simulink model "Longitudinal_old"  (R2025b)
settings: Solver=VariableStepAuto  StartTime=0.0  StopTime=100  RelTol=1e-3
undefined symbols (not defined in the file): car, m, R, Tau_1, Tau_2, Tau_3, Tau_4, Tau_EM, tyre
libraries: simulink x4
(part 1 of 2)
settings Model: Creator=mzacc  LastModifiedBy=giust

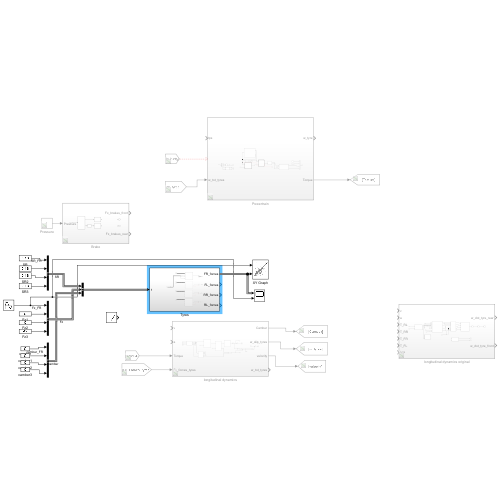
[thumbnail: Simulink's stored preview of the top-level diagram]
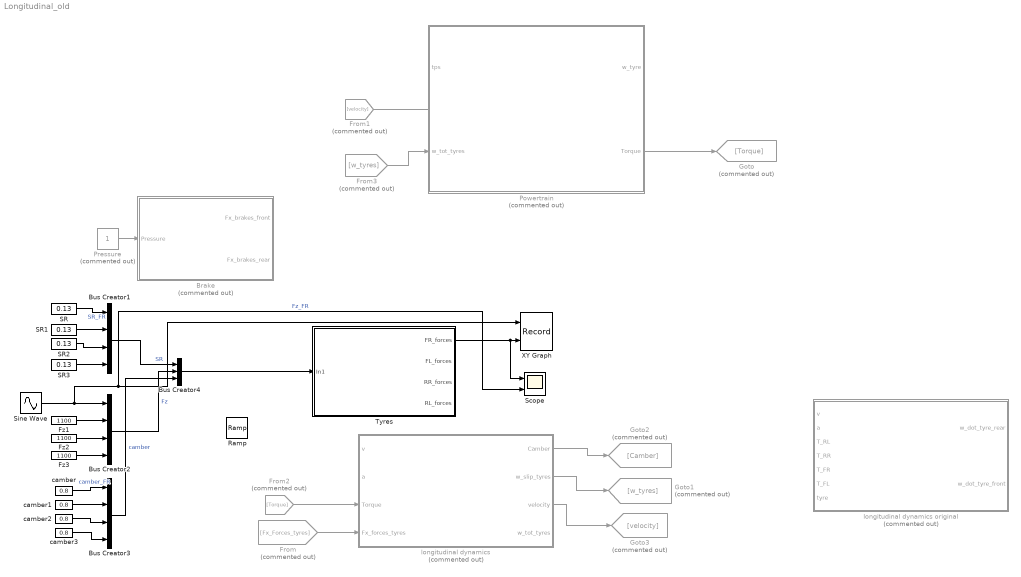
== system Longitudinal_old ==
  Brake : Subsystem  Commented=on
  Bus Creator1 : BusCreator  Inputs=4
  Bus Creator2 : BusCreator  Inputs=4
  Bus Creator3 : BusCreator  Inputs=4
  Bus Creator4 : BusCreator  Inputs=3
  From : From  Commented=on  GotoTag=Fx_Forces_tyres
  From1 : From  Commented=on  GotoTag=velocity
  From2 : From  Commented=on  GotoTag=Torque
  From3 : From  Commented=on  GotoTag=w_tyres
  Fz1 : Constant  Value=1100
  Fz2 : Constant  Value=1100
  Fz3 : Constant  Value=1100
  Goto : Goto  Commented=on  GotoTag=Torque
  Goto1 : Goto  Commented=on  GotoTag=w_tyres
  Goto2 : Goto  Commented=on  GotoTag=Camber
  Goto3 : Goto  Commented=on  GotoTag=velocity
  Powertrain : Subsystem  Commented=on
  Pressure : Constant  Commented=on
  Ramp : simulink/Sources/Ramp  slope=0.05  start=0  InitialOutput=-3
  SR{,1..3} (4 alike) : Constant  Value=0.13
  Scope : Scope  NumInputPorts=2
      settings: ActiveDisplayYMinimum=-298.14658012826334  ActiveDisplayYMaximum=2683.3192211543706
  Sine Wave : Sin  Amplitude=550  Bias=550  SampleTime=0
  Tyres : Subsystem
  XY Graph : Record  NumPorts=2.0  FileSettingsInternal="{\"entries\":[{\"content\":{\"excelSettings\":{\"content\":{},\"type\":\"Streamout.ExcelSettings\"},\"parquetSettings\":{\"content\":{},\"type\":\"Streamout.ParquetSettings\"}},\"type\":\"Streamout.FileSettingStorage\",\"uuid\":\"\"}],\"packageUris\":[\"http:\\/\\/schema.mathworks.com\\/mf0\\/streamout_blocks\\/R2020a\"],\"version\":\"1.0\"}"  FrameSettings=[0, 0]  Layout=[1 1]  SignalsInternal="{\"entries\":[{\"content\":{\"signals\":[{\"content\":{\"blockPath\":[],\"dimensions\":[1],\"domain\":\"\",\"lineColor\":\"#a2142f\",\"plots\":[ 1 ],\"port\":1,\"sid\":[\"\"],\"signalID\":1,\"signalName\":\"Fz_FR\"},\"type\":\"RecordBlkView.Signal\",\"uuid\":\"\"},{\"content\":{\"blockPath\":[],\"dimensions\":[1],\"domain\":\"\",\"hasChildren\":true,\"lineColor\":\"#4dbeee\",\"lineWidth\":2,\"port\":2,\"sid\":[\"\"],\"signalID\":2,\"signalName\":\"Tyres:1\"},\"type\":\"RecordBlkView.Signal\",\"uuid\":\"\"},{\"content\":{\"blockPath\":[],\"dimensions\":[1],\"domain\":\"\",\"leafPath\":\"Tyres:1.Fx_FR\",\"lineColor\":\"#7e2f8e\",\"lineWidth\":2,\"parentID\":2,\"plots\":[ 1 ],\"port\":2,\"sid\":[\"\"],\"signalID\":3,\"signalName\":\"Tyres:1.Fx_FR\"},\"type\":\"RecordBlkView.Signal\",\"uuid\":\"\"},{\"content\":{\"blockPath\":[],\"dimensions\":[1],\"domain\":\"\",\"leafPath\":\"Tyres:1.signal2\",\"lineColor\":\"#b746ff\",\"lineWidth\":2,\"parentID\":2,\"port\":2,\"sid\":[\"\"],\"signalID\":4,\"signalName\":\"Tyres:1.signal2\"},\"type\":\"RecordBlkView.Signal\",\"uuid\":\"\"}]},\"type\":\"RecordBlkView.InputSignals\",\"uuid\":\"\"}],\"packageUris\":[\"http:\\/\\/schema.mathworks.com\\/mf0\\/streamout_blocks\\/R2020a\"],\"version\":\"1.0\"}"  VisualizationBindings="{\"xyplotplugin\":{\"info\":[{\"series\":[{\"bindingParametersList\":[{\"parameter\":\"X-Axis\",\"signalID\":1,\"signalName\":\"Fz_FR\"},{\"parameter\":\"Y-Axis\",\"signalID\":3,\"signalName\":\"Tyres:1.Fx_FR\"},{\"parameter\":\"X-Axis\",\"signalID\":1,\"signalName\":\"Fz_FR\"},{\"parameter\":\"Y-Axis\",\"signalID\":3,\"signalName\":\"Tyres:1.Fx_FR\"}],\"seriesID\":0}],\"subplotID\":1}]}}"  CompatibilityTag=XY
  camber{,1..3} (4 alike) : Constant  Value=0.8
  longitudinal dynamics : Subsystem  Commented=on
  longitudinal dynamics original : Subsystem  Commented=on
  wires:
  Pressure/1 -> Brake/1(Pressure)
  From/1 -> longitudinal dynamics/4(Fx_forces_tyres)
  From2/1 -> longitudinal dynamics/3(Torque)
  Powertrain/2(Torque) -> Goto/1
  longitudinal dynamics/2(w_slip_tyres) -> Goto1/1
  longitudinal dynamics/1(Camber) -> Goto2/1
  longitudinal dynamics/3(velocity) -> Goto3/1
  From1/1 -> ?
  From3/1 -> Powertrain/2(w_tot_tyres)
  SR/1 -> Bus Creator1/1  "SR_FR"
  SR1/1 -> Bus Creator1/2
  SR2/1 -> Bus Creator1/3
  SR3/1 -> Bus Creator1/4
  Sine Wave/1 -> Scope/2, XY Graph/1, Bus Creator2/1  "Fz_FR"
  Fz1/1 -> Bus Creator2/2
  Fz2/1 -> Bus Creator2/3
  Fz3/1 -> Bus Creator2/4
  camber/1 -> Bus Creator3/1  "camber_FR"
  camber1/1 -> Bus Creator3/2
  camber2/1 -> Bus Creator3/3
  camber3/1 -> Bus Creator3/4
  Bus Creator1/1 -> Bus Creator4/1  "SR"
  Bus Creator2/1 -> Bus Creator4/2  "Fz"
  Bus Creator3/1 -> Bus Creator4/3  "camber"
  Bus Creator4/1 -> Tyres/1(In1)
  Tyres/1(FR_forces) -> Scope/1, XY Graph/2

== system Longitudinal_old/Brake ==
  Pressure : Inport
  Brake Balance : Subsystem
  Front Caliper : Subsystem
  Proportioning Valve : Subsystem
  Rear Caliper : Subsystem
  Fx_brakes_front : Outport
  Fx_brakes_rear : Outport  Port=2
  wires:
  Pressure/1 -> Brake Balance/1(In1)
  Brake Balance/1(P_Front) -> Front Caliper/1(P_Front)
  Proportioning Valve/1(p_rear_mod) -> Rear Caliper/1(P_rear)
  Brake Balance/2(P_rear) -> Proportioning Valve/1(P_rear)

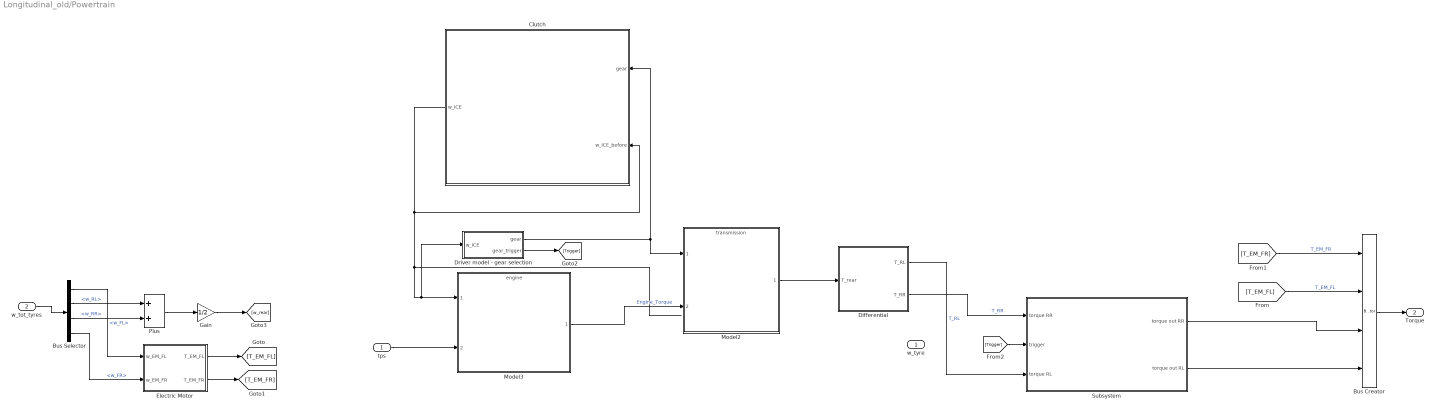
== system Longitudinal_old/Powertrain ==
  tps : Inport
  w_tot_tyres : Inport  Port=2
  Bus Creator : BusCreator  Inputs=4
  Bus Selector : BusSelector  OutputSignals=w_FL,w_RL,w_RR,w_FR
  Clutch : Subsystem
  Differential : Subsystem
  Driver model - gear selection : Subsystem
  Electric Motor : Subsystem
  Gain : Gain  Gain=1/2
  Model2 : ModelReference  ModelNameDialog=transmission.slx  SimulationMode=Normal  ModelReferenceVersion=3.9
  Model3 : ModelReference  ModelNameDialog=engine.slx  SimulationMode=Normal  ModelReferenceVersion=3.1
  Plus : Sum
  Subsystem : Subsystem
  w_tyre : Outport
  Torque : Outport  Port=2
  wires:
  Model3/1 -> Model2/2  "Engine_Torque"
  tps/1 -> Model3/2
  Model2/1 -> Differential/1(T_rear)
  ? -> w_tyre/1
  Bus Creator/1 -> Torque/1
  Electric Motor/1(T_EM_FL) -> [T_EM_FL]
  Electric Motor/2(T_EM_FR) -> [T_EM_FR]
  [T_EM_FL] -> Bus Creator/2  "T_EM_FL"
  [T_EM_FR] -> Bus Creator/1  "T_EM_FR"
  Differential/2(T_RR) -> Subsystem/1(torque RR)  "T_RR"
  Differential/1(T_RL) -> Subsystem/3(torque RL)  "T_RL"
  Subsystem/1(torque out RR) -> Bus Creator/3
  Subsystem/2(torque out RL) -> Bus Creator/4
  Driver model - gear selection/2(gear_trigger) -> [Trigger]
  [Trigger] -> Subsystem/2(trigger)
  w_tot_tyres/1 -> Bus Selector/1
  Bus Selector/1 -> Electric Motor/1(w_EM_FL)  "<w_FL>"
  Bus Selector/2 -> Plus/1  "<w_RL>"
  Bus Selector/4 -> Electric Motor/2(w_EM_FR)  "<w_FR>"
  Gain/1 -> [w_rear]
  Bus Selector/3 -> Plus/2  "<w_RR>"
  Plus/1 -> Gain/1
  Driver model - gear selection/1(gear) -> Clutch/1(gear), Model2/1
  Clutch/1(w_ICE) -> Clutch/2(w_ICE_before), Model3/1, Driver model - gear selection/1(w_ICE)

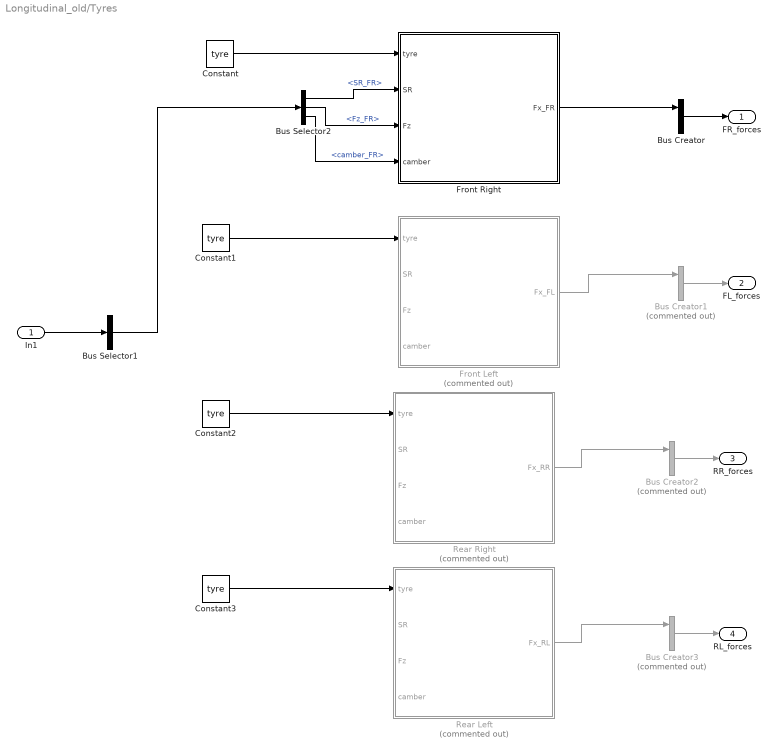
== system Longitudinal_old/Tyres ==
  In1 : Inport
  Bus Creator : BusCreator  Inputs=2
  Bus Creator1 : BusCreator  Commented=on  Inputs=2
  Bus Creator2 : BusCreator  Commented=on  Inputs=2
  Bus Creator3 : BusCreator  Commented=on  Inputs=2
  Bus Selector1 : BusSelector  OutputSignals=SR.SR_FR,Fz.Fz_FR,camber.camber_FR  OutputAsBus=on
  Bus Selector2 : BusSelector  OutputSignals=SR_FR,Fz_FR,camber_FR
  Constant{,1..3} (4 alike) : Constant  Value=tyre  OutDataTypeStr=Bus: slBus1
  Front Left : MATLAB Function  Commented=on  TreatAsAtomicUnit=on
  Front Right : MATLAB Function  TreatAsAtomicUnit=on
  Rear Left : MATLAB Function  Commented=on  TreatAsAtomicUnit=on
  Rear Right : MATLAB Function  Commented=on  TreatAsAtomicUnit=on
  FR_forces : Outport
  FL_forces : Outport  Port=2
  RR_forces : Outport  Port=3
  RL_forces : Outport  Port=4
  wires:
  Front Right/1(Fx_FR) -> Bus Creator/1
  Bus Creator/1 -> FR_forces/1
  Front Left/1(Fx_FL) -> Bus Creator1/1
  ? -> Bus Creator1/2
  Bus Creator1/1 -> FL_forces/1
  Rear Right/1(Fx_RR) -> Bus Creator2/1
  ? -> Bus Creator2/2
  Bus Creator2/1 -> RR_forces/1
  Rear Left/1(Fx_RL) -> Bus Creator3/1
  ? -> Bus Creator3/2
  Bus Creator3/1 -> RL_forces/1
  Constant/1 -> Front Right/1(tyre)
  Constant1/1 -> Front Left/1(tyre)
  Constant2/1 -> Rear Right/1(tyre)
  Constant3/1 -> Rear Left/1(tyre)
  In1/1 -> Bus Selector1/1
  Bus Selector1/1 -> Bus Selector2/1
  Bus Selector2/1 -> Front Right/2(SR)  "<SR_FR>"
  Bus Selector2/2 -> Front Right/3(Fz)  "<Fz_FR>"
  Bus Selector2/3 -> Front Right/4(camber)  "<camber_FR>"

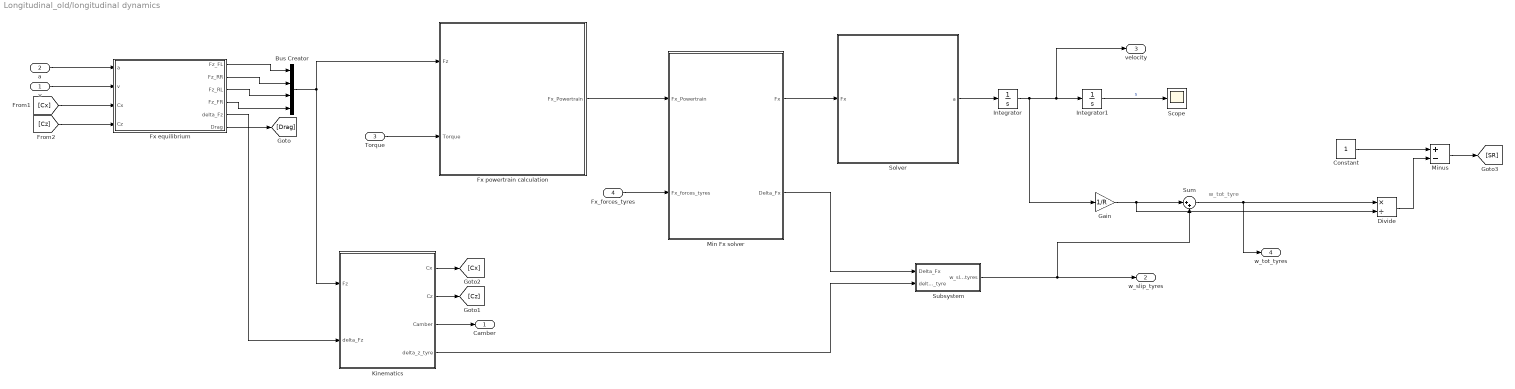
== system Longitudinal_old/longitudinal dynamics ==
  note: w_tot_tyre
  v : Inport
  a : Inport  Port=2
  Torque : Inport  Port=3
  Fx_forces_tyres : Inport  Port=4
  Bus Creator : BusCreator  Inputs=4
  Constant : Constant
  Divide : Product  Inputs=*/
  Fx equilibrium : MATLAB Function  TreatAsAtomicUnit=on
  Fx powertrain calculation : Subsystem
  Gain : Gain  Gain=1/R
  Integrator : Integrator
  Integrator1 : Integrator
  Kinematics : Subsystem
  Min Fx solver : Subsystem
  Minus : Sum  Inputs=+-
  Scope : Scope
  Solver : Subsystem
  Subsystem : Subsystem
  Sum : Sum  Inputs=|++
  Camber : Outport
  w_slip_tyres : Outport  Port=2
  velocity : Outport  Port=3
  w_tot_tyres : Outport  Port=4
  wires:
  a/1 -> Fx equilibrium/1(a)
  v/1 -> Fx equilibrium/2(v)
  Torque/1 -> Fx powertrain calculation/2(Torque)
  Integrator1/1 -> Scope/1  "s"
  Integrator/1 -> Gain/1, velocity/1, Integrator1/1
  Solver/1(a) -> Integrator/1
  Fx equilibrium/1(Fz_FL) -> Bus Creator/1
  Fx equilibrium/2(Fz_RR) -> Bus Creator/2
  Fx equilibrium/3(Fz_RL) -> Bus Creator/3
  Fx equilibrium/4(Fz_FR) -> Bus Creator/4
  Bus Creator/1 -> Kinematics/1(Fz), Fx powertrain calculation/1(Fz)
  Fx powertrain calculation/1(Fx_Powertrain) -> Min Fx solver/1(Fx_Powertrain)
  Fx_forces_tyres/1 -> Min Fx solver/2(Fx_forces_tyres)
  Min Fx solver/1(Fx) -> Solver/1(Fx)
  Min Fx solver/2(Delta_Fx) -> Subsystem/1(Delta_Fx)
  Kinematics/4(delta_z_tyre) -> Subsystem/2(delta_z_tyre)
  Kinematics/3(Camber) -> Camber/1
  Subsystem/1(w_slip_tyres) -> Sum/2, w_slip_tyres/1
  Fx equilibrium/6(Drag) -> [Drag]
  Fx equilibrium/5(delta_Fz) -> Kinematics/2(delta_Fz)
  Kinematics/2(Cz) -> [Cz]
  Kinematics/1(Cx) -> [Cx]
  [Cx] -> Fx equilibrium/3(Cx)
  [Cz] -> Fx equilibrium/4(Cz)
  Gain/1 -> Divide/2, Sum/1
  Sum/1 -> w_tot_tyres/1, Divide/1
  Constant/1 -> Minus/1
  Divide/1 -> Minus/2
  Minus/1 -> [SR]

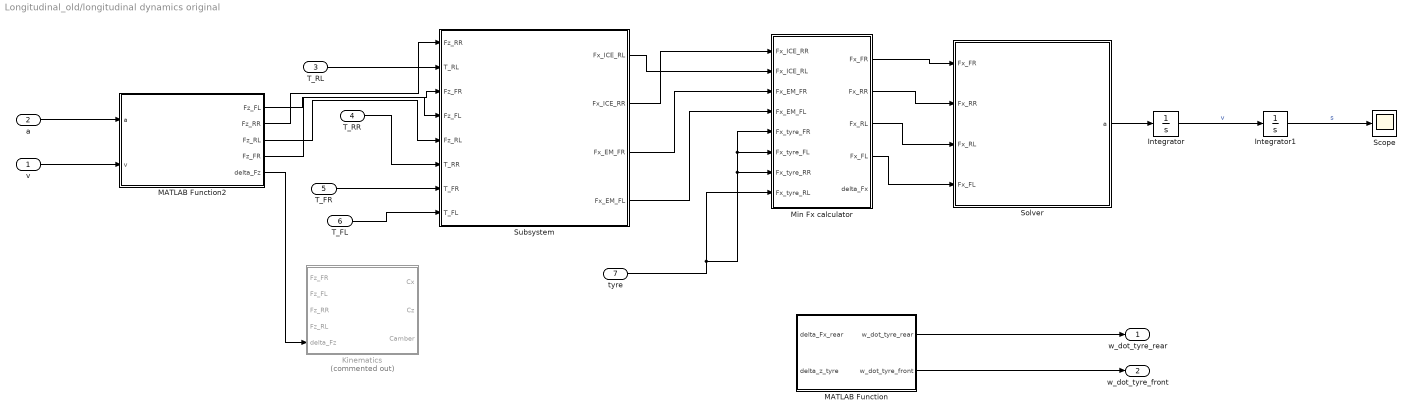
== system Longitudinal_old/longitudinal dynamics original ==
  v : Inport
  a : Inport  Port=2
  T_RL : Inport  Port=3
  T_RR : Inport  Port=4
  T_FR : Inport  Port=5
  T_FL : Inport  Port=6
  tyre : Inport  Port=7
  Integrator : Integrator
  Integrator1 : Integrator
  Kinematics : Subsystem  Commented=on
  MATLAB Function : MATLAB Function  TreatAsAtomicUnit=on
  MATLAB Function2 : MATLAB Function  TreatAsAtomicUnit=on
  Min Fx calculator : MATLAB Function  TreatAsAtomicUnit=on
  Scope : Scope
  Solver : Subsystem
  Subsystem : Subsystem
  w_dot_tyre_rear : Outport
  w_dot_tyre_front : Outport  Port=2
  wires:
  a/1 -> MATLAB Function2/1(a)
  v/1 -> MATLAB Function2/2(v)
  T_RL/1 -> Subsystem/2(T_RL)
  T_RR/1 -> Subsystem/6(T_RR)
  T_FR/1 -> Subsystem/7(T_FR)
  T_FL/1 -> Subsystem/8(T_FL)
  MATLAB Function2/4(Fz_FR) -> Subsystem/3(Fz_FR)
  MATLAB Function2/3(Fz_RL) -> Subsystem/5(Fz_RL)
  MATLAB Function2/2(Fz_RR) -> Subsystem/1(Fz_RR)
  MATLAB Function2/1(Fz_FL) -> Subsystem/4(Fz_FL)
  Subsystem/1(Fx_ICE_RL) -> Min Fx calculator/2(Fx_ICE_RL)
  Subsystem/2(Fx_ICE_RR) -> Min Fx calculator/1(Fx_ICE_RR)
  Subsystem/3(Fx_EM_FR) -> Min Fx calculator/3(Fx_EM_FR)
  Subsystem/4(Fx_EM_FL) -> Min Fx calculator/4(Fx_EM_FL)
  tyre/1 -> Min Fx calculator/6(Fx_tyre_FL), Min Fx calculator/5(Fx_tyre_FR), Min Fx calculator/7(Fx_tyre_RR), Min Fx calculator/8(Fx_tyre_RL)
  Integrator1/1 -> Scope/1  "s"
  Integrator/1 -> Integrator1/1  "v"
  Solver/1(a) -> Integrator/1
  Min Fx calculator/1(Fx_FR) -> Solver/1(Fx_FR)
  Min Fx calculator/2(Fx_RR) -> Solver/2(Fx_RR)
  Min Fx calculator/3(Fx_RL) -> Solver/3(Fx_RL)
  Min Fx calculator/4(Fx_FL) -> Solver/4(Fx_FL)
  MATLAB Function2/5(delta_Fz) -> Kinematics/5(delta_Fz)
  MATLAB Function/1(w_dot_tyre_rear) -> w_dot_tyre_rear/1
  MATLAB Function/2(w_dot_tyre_front) -> w_dot_tyre_front/1

== system Longitudinal_old/Brake/Brake Balance ==
  In1 : Inport
  Gain : Gain  Gain=car.brakebalance
  Gain1 : Gain  Gain=1-car.brakebalance
  P_Front : Outport
  P_rear : Outport  Port=2
  wires:
  In1/1 -> Gain1/1, Gain/1
  Gain1/1 -> P_rear/1  "P_rear"
  Gain/1 -> P_Front/1  "P_Front"

== system Longitudinal_old/Brake/Front Caliper ==
  P_Front : Inport
  Gain : Gain  Gain=4
  Pad Friction : Gain  Gain=car.brakepad_friction_coeff
  Piston Area : Gain  Gain=pi*(car.brakepistondiameter)^2/4
  Out1 : Outport
  wires:
  P_Front/1 -> Gain/1
  Gain/1 -> Piston Area/1
  Piston Area/1 -> Pad Friction/1
  Pad Friction/1 -> Out1/1

== system Longitudinal_old/Brake/Proportioning Valve ==
  P_rear : Inport
  Saturation : Saturate  UpperLimit=car.proportioning_valve_cutting_p  LowerLimit=0
  p_rear_mod : Outport
  wires:
  Saturation/1 -> p_rear_mod/1
  P_rear/1 -> Saturation/1

== system Longitudinal_old/Brake/Rear Caliper ==
  P_rear : Inport
  Gain : Gain  Gain=4
  Pad Friction : Gain  Gain=car.brakepad_friction_coeff
  Piston Area : Gain  Gain=pi*(car.brakepistondiameter)^2/4
  Out1 : Outport
  wires:
  Piston Area/1 -> Pad Friction/1
  Gain/1 -> Piston Area/1
  P_rear/1 -> Gain/1
  Pad Friction/1 -> Out1/1

== system Longitudinal_old/Powertrain/Clutch ==
  gear : Inport
  w_ICE_before : Inport  Port=2
  1-D Lookup Table1 : Lookup_n-D  NumberOfTableDimensions=1  BreakpointsForDimension1=[0;1;2;3;4]  Table=[Tau_1; Tau_2; Tau_3; Tau_4]  InternalRulePriority=Speed  RndMeth=Simplest
  Add : Sum  Inputs=+++
  Delay One Step : Delay  DelayLength=1
  Gain1 : Gain  Gain=0
  Product : Product
  Ramp : simulink/Sources/Ramp  slope=-car.clutch.RPM.start/car.clutch.time.engaged  start=0  InitialOutput=car.clutch.RPM.start
  Saturation : Saturate  UpperLimit=car.initialconditions.EngineRPM  LowerLimit=0
  w_ICE : Outport
  wires:
  Saturation/1 -> Add/1
  Ramp/1 -> Saturation/1
  [w_rear] -> Product/2
  1-D Lookup Table1/1 -> Product/1
  Product/1 -> Add/3
  Delay One Step/1 -> Gain1/1
  w_ICE_before/1 -> Delay One Step/1
  gear/1 -> 1-D Lookup Table1/1
  Gain1/1 -> Add/2
  Add/1 -> w_ICE/1  "0"

== system Longitudinal_old/Powertrain/Differential ==
  T_rear : Inport
  Gain : Gain  Gain=0.5
  T_RL : Outport
  T_RR : Outport  Port=2
  wires:
  T_rear/1 -> Gain/1
  Gain/1 -> T_RR/1, T_RL/1

== system Longitudinal_old/Powertrain/Driver model - gear selection ==
  w_ICE : Inport
  MATLAB Function3 : MATLAB Function  TreatAsAtomicUnit=on
  Unit Delay : UnitDelay  InitialCondition=2  SampleTime=-1  HasFrameUpgradeWarning=on
  gear : Outport
  gear_trigger : Outport  Port=2
  wires:
  MATLAB Function3/2(gear_out) -> gear/1, Unit Delay/1
  w_ICE/1 -> MATLAB Function3/1(w_ICE)
  Unit Delay/1 -> MATLAB Function3/2(gear_in)
  MATLAB Function3/1(gear_trigger) -> gear_trigger/1  "trigger"

== system Longitudinal_old/Powertrain/Electric Motor ==
  w_EM_FL : Inport
  w_EM_FR : Inport  Port=2
  EM torque LUT : Lookup_n-D  NumberOfTableDimensions=1  BreakpointsForDimension1=[0;5415.9399999999996;5455.8699999999999;5494.6300000000001;5524.8000000000002;5801.2200000000003;6194.8599999999997;6620.2799999999997;6996.5;7478.6599999999999;8072.5500000000002;8891.9799999999996;8998.9200000000001;9966.8600000000006;10994.200000000001;11872.6;13016.16;13972.65;15994.85]  Table=[6.914188214;6.910217161;6.868869365;6.845730801;6.823144351;6.614154423;6.313463369;6.000782967;5.723209117;5.399066491;4.994963902;4.498183933;4.450257084;3.941031953;3.525109858;3.198600505;2.816719111;2.558901053;2.040423041]  InternalRulePriority=Speed  RndMeth=Simplest
  EM torque LUT1 : Lookup_n-D  NumberOfTableDimensions=1  BreakpointsForDimension1=[0;5415.9399999999996;5455.8699999999999;5494.6300000000001;5524.8000000000002;5801.2200000000003;6194.8599999999997;6620.2799999999997;6996.5;7478.6599999999999;8072.5500000000002;8891.9799999999996;8998.9200000000001;9966.8600000000006;10994.200000000001;11872.6;13016.16;13972.65;15994.85]  Table=[6.914188214;6.910217161;6.868869365;6.845730801;6.823144351;6.614154423;6.313463369;6.000782967;5.723209117;5.399066491;4.994963902;4.498183933;4.450257084;3.941031953;3.525109858;3.198600505;2.816719111;2.558901053;2.040423041]  InternalRulePriority=Speed  RndMeth=Simplest
  Gain : Gain  Gain=Tau_EM
  Gain1 : Gain  Gain=Tau_EM
  T_EM_FL : Outport
  T_EM_FR : Outport  Port=2
  wires:
  EM torque LUT/1 -> Gain/1
  w_EM_FL/1 -> EM torque LUT/1
  Gain1/1 -> T_EM_FR/1
  w_EM_FR/1 -> EM torque LUT1/1
  EM torque LUT1/1 -> Gain1/1
  Gain/1 -> T_EM_FL/1

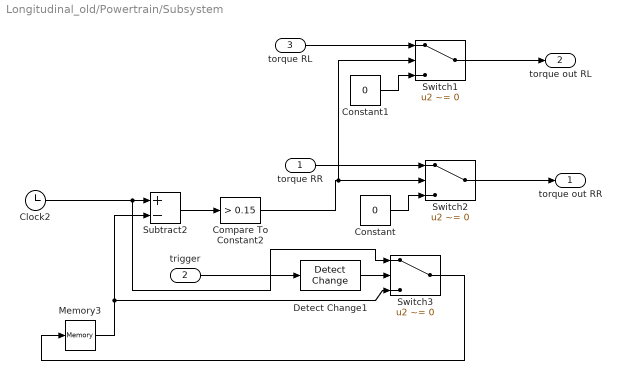
== system Longitudinal_old/Powertrain/Subsystem ==
  torque RR : Inport
  trigger : Inport  Port=2
  torque RL : Inport  Port=3
  Clock2 : Clock
  Compare To Constant2 : simulink/Logic and Bit Operations/Compare To Constant  relop=>  const=0.15  OutDataTypeStr=boolean
  Constant : Constant  Value=0
  Constant1 : Constant  Value=0
  Detect Change1 : simulink/Logic and Bit Operations/Detect Change  vinit=0  OutDataTypeStr=boolean
  Memory3 : Memory
  Subtract2 : Sum  Inputs=+-
  Switch1 : Switch  Criteria=u2 ~= 0  SaturateOnIntegerOverflow=off  InputSameDT=off
  Switch2 : Switch  Criteria=u2 ~= 0  SaturateOnIntegerOverflow=off  InputSameDT=off
  Switch3 : Switch  Criteria=u2 ~= 0  SaturateOnIntegerOverflow=off  InputSameDT=off
  torque out RR : Outport
  torque out RL : Outport  Port=2
  wires:
  Memory3/1 -> Switch3/3, Subtract2/2
  Detect Change1/1 -> Switch3/2
  trigger/1 -> Detect Change1/1
  Constant/1 -> Switch2/3
  Clock2/1 -> Switch3/1, Subtract2/1
  Switch3/1 -> Memory3/1
  Subtract2/1 -> Compare To Constant2/1
  Switch2/1 -> torque out RR/1
  torque RR/1 -> Switch2/1
  torque RL/1 -> Switch1/1
  Switch1/1 -> torque out RL/1
  Compare To Constant2/1 -> Switch1/2, Switch2/2
  Constant1/1 -> Switch1/3

== system Longitudinal_old/longitudinal dynamics/Fx powertrain calculation ==
  Fz : Inport
  Torque : Inport  Port=2
  Bus Creator : BusCreator  Inputs=4
  Bus Selector : BusSelector  OutputSignals=Fz_FL,Fz_RR,Fz_RL,Fz_FR
  Bus Selector1 : BusSelector  OutputSignals=T_EM_FR,T_EM_FL,T_RL,T_RR
  FL : MATLAB Function  TreatAsAtomicUnit=on
  FR : MATLAB Function  TreatAsAtomicUnit=on
  RL : MATLAB Function  TreatAsAtomicUnit=on
  RR : MATLAB Function  TreatAsAtomicUnit=on
  Fx_Powertrain : Outport
  wires:
  Fz/1 -> Bus Selector/1
  Torque/1 -> Bus Selector1/1
  Bus Selector/1 -> FL/1(Fz)  "<Fz_FL>"
  Bus Selector1/2 -> FL/2(T)  "<T_EM_FL>"
  Bus Selector/2 -> RR/1(Fz)  "<Fz_RR>"
  Bus Selector1/4 -> RR/2(T)  "<T_RR>"
  Bus Selector/3 -> RL/1(Fz)  "<Fz_RL>"
  Bus Selector/4 -> FR/1(Fz)  "<Fz_FR>"
  Bus Selector1/1 -> FR/2(T)  "<T_EM_FR>"
  Bus Selector1/3 -> RL/2(T)  "<T_RL>"
  FL/1(Fx_EM_FL) -> Bus Creator/1
  RR/1(Fx_ICE_RR) -> Bus Creator/2
  FR/1(Fx_EM_FR) -> Bus Creator/3
  RL/1(Fx_ICE_RL) -> Bus Creator/4
  Bus Creator/1 -> Fx_Powertrain/1

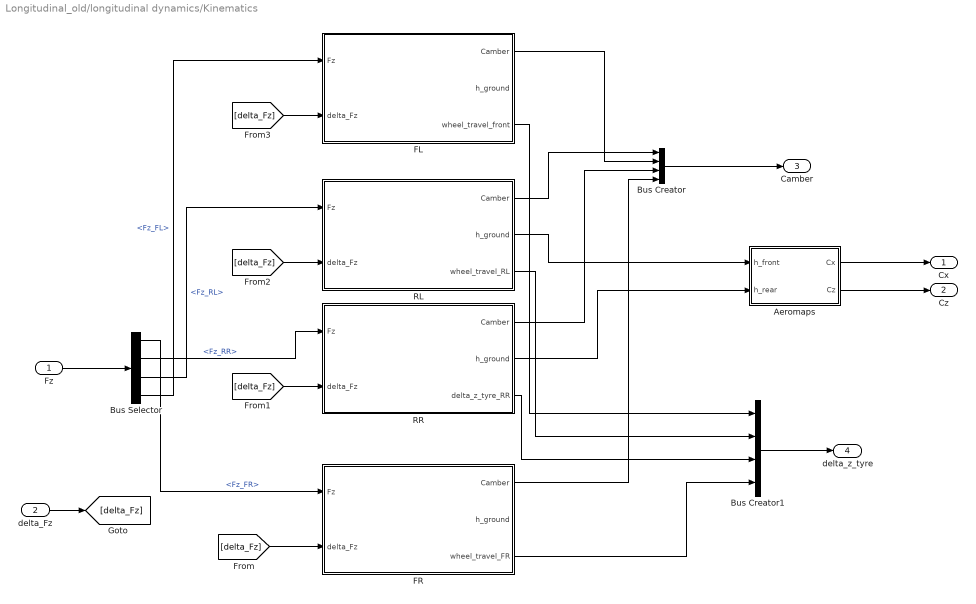
== system Longitudinal_old/longitudinal dynamics/Kinematics ==
  Fz : Inport
  delta_Fz : Inport  Port=2
  Aeromaps : Subsystem
  Bus Creator : BusCreator  Inputs=4
  Bus Creator1 : BusCreator  Inputs=4
  Bus Selector : BusSelector  OutputSignals=Fz_FR,Fz_RR,Fz_RL,Fz_FL
  FL : Subsystem
  FR : Subsystem
  RL : Subsystem
  RR : Subsystem
  Cx : Outport
  Cz : Outport  Port=2
  Camber : Outport  Port=3
  delta_z_tyre : Outport  Port=4
  wires:
  Aeromaps/1(Cx) -> Cx/1
  Aeromaps/2(Cz) -> Cz/1
  FL/1(Camber) -> Bus Creator/2
  RR/1(Camber) -> Bus Creator/3
  FR/1(Camber) -> Bus Creator/4
  RL/2(h_ground) -> Aeromaps/1(h_front)
  RR/2(h_ground) -> Aeromaps/2(h_rear)
  RL/1(Camber) -> Bus Creator/1
  Bus Creator/1 -> Camber/1
  Fz/1 -> Bus Selector/1
  Bus Selector/1 -> FR/1(Fz)  "<Fz_FR>"
  Bus Selector/2 -> RR/1(Fz)  "<Fz_RR>"
  Bus Selector/3 -> RL/1(Fz)  "<Fz_RL>"
  Bus Selector/4 -> FL/1(Fz)  "<Fz_FL>"
  [delta_Fz] -> FR/2(delta_Fz)
  [delta_Fz] -> RR/2(delta_Fz)
  [delta_Fz] -> RL/2(delta_Fz)
  [delta_Fz] -> FL/2(delta_Fz)
  Bus Creator1/1 -> delta_z_tyre/1
  FR/3(wheel_travel_FR) -> Bus Creator1/4
  RR/3(delta_z_tyre_RR) -> Bus Creator1/3
  RL/3(wheel_travel_RL) -> Bus Creator1/2
  FL/3(wheel_travel_front) -> Bus Creator1/1
  delta_Fz/1 -> [delta_Fz]

== system Longitudinal_old/longitudinal dynamics/Min Fx solver ==
  Fx_Powertrain : Inport
  Fx_forces_tyres : Inport  Port=2
  Bus Creator : BusCreator  Inputs=4
  Bus Creator1 : BusCreator  Inputs=4
  Bus Selector : BusSelector  OutputSignals=Fx_ICE_RR,Fx_ICE_RL,Fx_EM_FL,Fx_EM_FR
  Bus Selector1 : BusSelector  OutputSignals=Fx_RL,Fx_RR,Fx_FR,Fx_FL
  FL : MATLAB Function  TreatAsAtomicUnit=on
  FR : MATLAB Function  TreatAsAtomicUnit=on
  RL : MATLAB Function  TreatAsAtomicUnit=on
  RR : MATLAB Function  TreatAsAtomicUnit=on
  Fx : Outport
  Delta_Fx : Outport  Port=2
  wires:
  Fx_Powertrain/1 -> Bus Selector/1
  Fx_forces_tyres/1 -> Bus Selector1/1
  Bus Selector/1 -> RR/1(Fx_ICE)  "<Fx_ICE_RR>"
  Bus Selector1/1 -> RL/2(Fx_tyre)  "<Fx_RL>"
  Bus Selector1/2 -> RR/2(Fx_tyre)  "<Fx_RR>"
  Bus Selector/2 -> RL/1(Fx_ICE)  "<Fx_ICE_RL>"
  RR/1(Fx_RR) -> Bus Creator/1
  RL/1(Fx_RL) -> Bus Creator/2
  Bus Creator/1 -> Fx/1
  Bus Selector1/4 -> FL/2(Fx_tyre)  "<Fx_FL>"
  Bus Selector1/3 -> FR/2(Fx_tyre)  "<Fx_FR>"
  Bus Selector/4 -> FR/1(Fx_EM)  "<Fx_EM_FR>"
  Bus Selector/3 -> FL/1(Fx_EM)  "<Fx_EM_FL>"
  FR/1(Fx_FR) -> Bus Creator/3
  FL/1(Fx_FL) -> Bus Creator/4
  Bus Creator1/1 -> Delta_Fx/1
  RR/2(delta_Fx_RR) -> Bus Creator1/1
  RL/2(delta_Fx_RL) -> Bus Creator1/2
  FR/2(delta_Fx_FR) -> Bus Creator1/3
  FL/2(delta_Fx_FL) -> Bus Creator1/4

== system Longitudinal_old/longitudinal dynamics/Solver ==
  Fx : Inport
  Add : Sum  Inputs=++++
  Bus Selector : BusSelector  OutputSignals=Fx_RR,Fx_RL,Fx_FR,Fx_FL
  Gain : Gain  Gain=1/m
  Subtract : Sum  Inputs=+-
  a : Outport
  wires:
  Add/1 -> Subtract/1
  Subtract/1 -> Gain/1
  [Drag] -> Subtract/2
  Gain/1 -> a/1  "a"
  Fx/1 -> Bus Selector/1
  Bus Selector/1 -> Add/1  "<Fx_RR>"
  Bus Selector/2 -> Add/2  "<Fx_RL>"
  Bus Selector/3 -> Add/3  "<Fx_FR>"
  Bus Selector/4 -> Add/4  "<Fx_FL>"

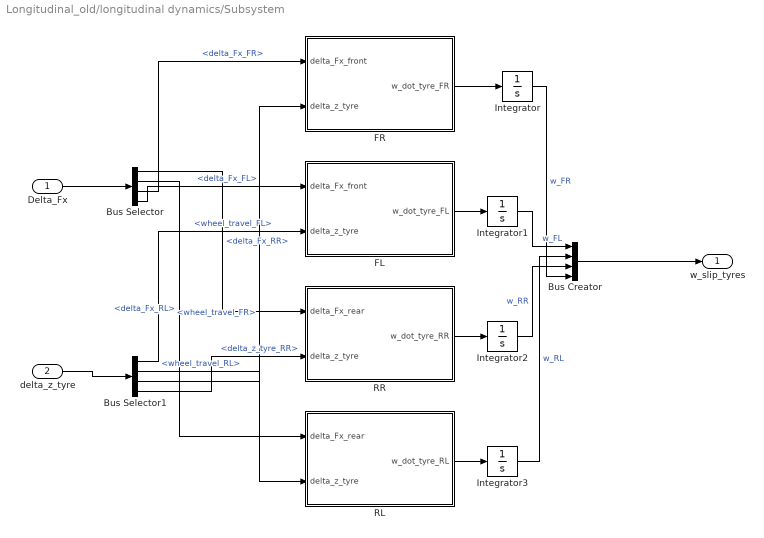
== system Longitudinal_old/longitudinal dynamics/Subsystem ==
  Delta_Fx : Inport
  delta_z_tyre : Inport  Port=2
  Bus Creator : BusCreator  Inputs=4
  Bus Selector : BusSelector  OutputSignals=delta_Fx_RR,delta_Fx_RL,delta_Fx_FR,delta_Fx_FL
  Bus Selector1 : BusSelector  OutputSignals=wheel_travel_FL,wheel_travel_RL,wheel_travel_FR,delta_z_tyre_RR
  FL : MATLAB Function  TreatAsAtomicUnit=on
  FR : MATLAB Function  TreatAsAtomicUnit=on
  Integrator{,1..3} (4 alike) : Integrator
  RL : MATLAB Function  TreatAsAtomicUnit=on
  RR : MATLAB Function  TreatAsAtomicUnit=on
  w_slip_tyres : Outport
  wires:
  Delta_Fx/1 -> Bus Selector/1
  delta_z_tyre/1 -> Bus Selector1/1
  Bus Selector/1 -> RR/1(delta_Fx_rear)  "<delta_Fx_RR>"
  Bus Selector/2 -> RL/1(delta_Fx_rear)  "<delta_Fx_RL>"
  Bus Selector/3 -> FR/1(delta_Fx_front)  "<delta_Fx_FR>"
  Bus Selector/4 -> FL/1(delta_Fx_front)  "<delta_Fx_FL>"
  Bus Selector1/1 -> FL/2(delta_z_tyre)  "<wheel_travel_FL>"
  Bus Selector1/2 -> RL/2(delta_z_tyre)  "<wheel_travel_RL>"
  Bus Selector1/4 -> RR/2(delta_z_tyre)  "<delta_z_tyre_RR>"
  Bus Selector1/3 -> FR/2(delta_z_tyre)  "<wheel_travel_FR>"
  Bus Creator/1 -> w_slip_tyres/1
  FR/1(w_dot_tyre_FR) -> Integrator/1
  Integrator/1 -> Bus Creator/4  "w_FR"
  FL/1(w_dot_tyre_FL) -> Integrator1/1
  Integrator1/1 -> Bus Creator/1  "w_FL"
  RR/1(w_dot_tyre_RR) -> Integrator2/1
  Integrator2/1 -> Bus Creator/3  "w_RR"
  RL/1(w_dot_tyre_RL) -> Integrator3/1
  Integrator3/1 -> Bus Creator/2  "w_RL"

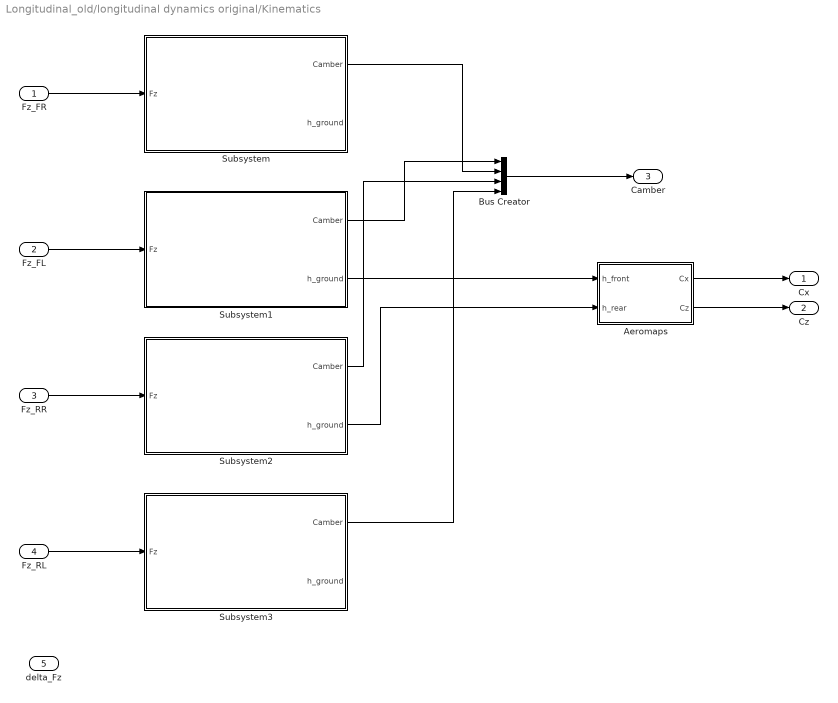
== system Longitudinal_old/longitudinal dynamics original/Kinematics ==
  Fz_FR : Inport
  Fz_FL : Inport  Port=2
  Fz_RR : Inport  Port=3
  Fz_RL : Inport  Port=4
  delta_Fz : Inport  Port=5
  Aeromaps : Subsystem
  Bus Creator : BusCreator  Inputs=4
  Subsystem : Subsystem
  Subsystem1 : Subsystem
  Subsystem2 : Subsystem
  Subsystem3 : Subsystem
  Cx : Outport
  Cz : Outport  Port=2
  Camber : Outport  Port=3
  wires:
  Aeromaps/1(Cx) -> Cx/1
  Aeromaps/2(Cz) -> Cz/1
  Fz_FR/1 -> Subsystem/1(Fz)
  Subsystem/1(Camber) -> Bus Creator/2
  Fz_FL/1 -> Subsystem1/1(Fz)
  Fz_RR/1 -> Subsystem2/1(Fz)
  Subsystem2/1(Camber) -> Bus Creator/3
  Subsystem3/1(Camber) -> Bus Creator/4
  Fz_RL/1 -> Subsystem3/1(Fz)
  Subsystem1/2(h_ground) -> Aeromaps/1(h_front)
  Subsystem2/2(h_ground) -> Aeromaps/2(h_rear)
  Subsystem1/1(Camber) -> Bus Creator/1
  Bus Creator/1 -> Camber/1

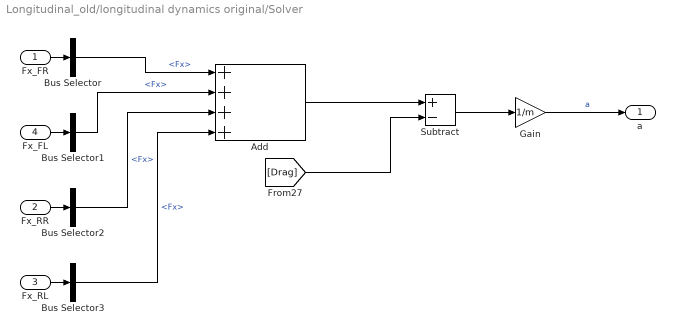
== system Longitudinal_old/longitudinal dynamics original/Solver ==
  Fx_FR : Inport
  Fx_RR : Inport  Port=2
  Fx_RL : Inport  Port=3
  Fx_FL : Inport  Port=4
  Add : Sum  Inputs=++++
  Bus Selector{,1..3} (4 alike) : BusSelector  OutputSignals=Fx
  Gain : Gain  Gain=1/m
  Subtract : Sum  Inputs=+-
  a : Outport
  wires:
  Add/1 -> Subtract/1
  Subtract/1 -> Gain/1
  [Drag] -> Subtract/2
  Gain/1 -> a/1  "a"
  Fx_FL/1 -> Bus Selector1/1
  Fx_RR/1 -> Bus Selector2/1
  Fx_RL/1 -> Bus Selector3/1
  Fx_FR/1 -> Bus Selector/1
  Bus Selector/1 -> Add/1  "<Fx>"
  Bus Selector1/1 -> Add/2  "<Fx>"
  Bus Selector2/1 -> Add/3  "<Fx>"
  Bus Selector3/1 -> Add/4  "<Fx>"

== system Longitudinal_old/longitudinal dynamics original/Subsystem ==
  Fz_RR : Inport
  T_RL : Inport  Port=2
  Fz_FR : Inport  Port=3
  Fz_FL : Inport  Port=4
  Fz_RL : Inport  Port=5
  T_RR : Inport  Port=6
  T_FR : Inport  Port=7
  T_FL : Inport  Port=8
  MATLAB Function : MATLAB Function  TreatAsAtomicUnit=on
  Fx_ICE_RL : Outport
  Fx_ICE_RR : Outport  Port=2
  Fx_EM_FR : Outport  Port=3
  Fx_EM_FL : Outport  Port=4

== system Longitudinal_old/longitudinal dynamics/Kinematics/Aeromaps ==
  h_front : Inport
  h_rear : Inport  Port=2
  Cx : Outport
  Cz : Outport  Port=2
  wires:
  h_front/1 -> Cx/1

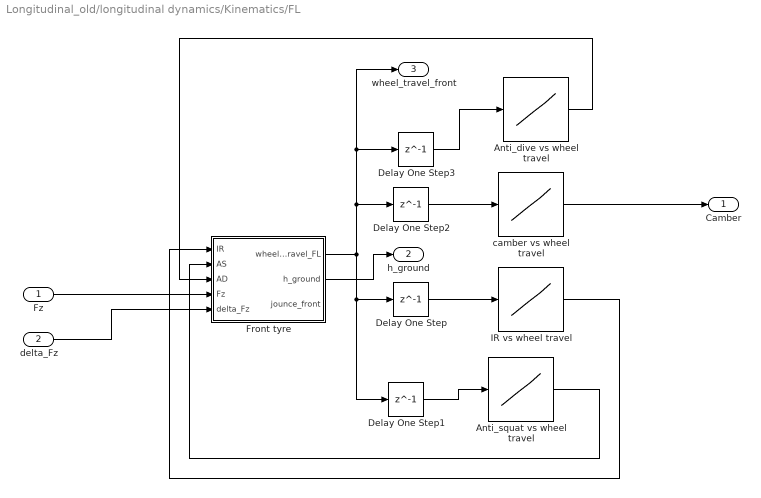
== system Longitudinal_old/longitudinal dynamics/Kinematics/FL ==
  Fz : Inport
  delta_Fz : Inport  Port=2
  Anti_dive vs wheel travel : Lookup_n-D  NumberOfTableDimensions=1  BreakpointsForDimension1=[-5:5]  Table=tanh([-5:5])  InternalRulePriority=Speed  RndMeth=Simplest
  Anti_squat vs wheel travel : Lookup_n-D  NumberOfTableDimensions=1  BreakpointsForDimension1=[-5:5]  Table=tanh([-5:5])  InternalRulePriority=Speed  RndMeth=Simplest
  Delay One Step{,1..3} (4 alike) : Delay  DelayLength=1
  Front tyre : MATLAB Function  TreatAsAtomicUnit=on
  IR vs wheel travel : Lookup_n-D  NumberOfTableDimensions=1  BreakpointsForDimension1=[-5:5]  Table=tanh([-5:5])  InternalRulePriority=Speed  RndMeth=Simplest
  camber vs wheel travel : Lookup_n-D  NumberOfTableDimensions=1  BreakpointsForDimension1=[-5:5]  Table=tanh([-5:5])  InternalRulePriority=Speed  RndMeth=Simplest
  Camber : Outport
  h_ground : Outport  Port=2
  wheel_travel_front : Outport  Port=3
  wires:
  Delay One Step2/1 -> camber vs wheel travel/1
  Front tyre/1(wheel_travel_FL) -> Delay One Step3/1, wheel_travel_front/1, Delay One Step2/1, Delay One Step1/1, Delay One Step/1
  Delay One Step/1 -> IR vs wheel travel/1
  camber vs wheel travel/1 -> Camber/1
  Anti_squat vs wheel travel/1 -> Front tyre/2(AS)
  IR vs wheel travel/1 -> Front tyre/1(IR)
  Delay One Step1/1 -> Anti_squat vs wheel travel/1
  Front tyre/2(h_ground) -> h_ground/1
  Fz/1 -> Front tyre/4(Fz)
  delta_Fz/1 -> Front tyre/5(delta_Fz)
  Delay One Step3/1 -> Anti_dive vs wheel travel/1
  Anti_dive vs wheel travel/1 -> Front tyre/3(AD)

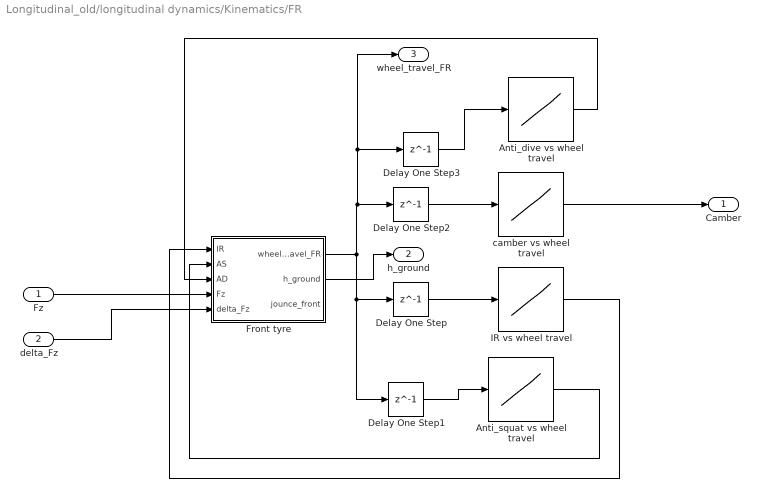
== system Longitudinal_old/longitudinal dynamics/Kinematics/FR ==
  Fz : Inport
  delta_Fz : Inport  Port=2
  Anti_dive vs wheel travel : Lookup_n-D  NumberOfTableDimensions=1  BreakpointsForDimension1=[-5:5]  Table=tanh([-5:5])  InternalRulePriority=Speed  RndMeth=Simplest
  Anti_squat vs wheel travel : Lookup_n-D  NumberOfTableDimensions=1  BreakpointsForDimension1=[-5:5]  Table=tanh([-5:5])  InternalRulePriority=Speed  RndMeth=Simplest
  Delay One Step{,1..3} (4 alike) : Delay  DelayLength=1
  Front tyre : MATLAB Function  TreatAsAtomicUnit=on
  IR vs wheel travel : Lookup_n-D  NumberOfTableDimensions=1  BreakpointsForDimension1=[-5:5]  Table=tanh([-5:5])  InternalRulePriority=Speed  RndMeth=Simplest
  camber vs wheel travel : Lookup_n-D  NumberOfTableDimensions=1  BreakpointsForDimension1=[-5:5]  Table=tanh([-5:5])  InternalRulePriority=Speed  RndMeth=Simplest
  Camber : Outport
  h_ground : Outport  Port=2
  wheel_travel_FR : Outport  Port=3
  wires:
  Delay One Step2/1 -> camber vs wheel travel/1
  Front tyre/1(wheel_travel_FR) -> Delay One Step3/1, wheel_travel_FR/1, Delay One Step2/1, Delay One Step1/1, Delay One Step/1
  Delay One Step/1 -> IR vs wheel travel/1
  camber vs wheel travel/1 -> Camber/1
  Anti_squat vs wheel travel/1 -> Front tyre/2(AS)
  IR vs wheel travel/1 -> Front tyre/1(IR)
  Delay One Step1/1 -> Anti_squat vs wheel travel/1
  Front tyre/2(h_ground) -> h_ground/1
  Fz/1 -> Front tyre/4(Fz)
  delta_Fz/1 -> Front tyre/5(delta_Fz)
  Anti_dive vs wheel travel/1 -> Front tyre/3(AD)
  Delay One Step3/1 -> Anti_dive vs wheel travel/1

== system Longitudinal_old/longitudinal dynamics/Kinematics/RL ==
  Fz : Inport
  delta_Fz : Inport  Port=2
  Anti_squat vs wheel travel : Lookup_n-D  NumberOfTableDimensions=1  BreakpointsForDimension1=[-5:5]  Table=tanh([-5:5])  InternalRulePriority=Speed  RndMeth=Simplest
  Delay One Step : Delay  DelayLength=1
  Delay One Step1 : Delay  DelayLength=1
  Delay One Step2 : Delay  DelayLength=1
  IR vs wheel travel : Lookup_n-D  NumberOfTableDimensions=1  BreakpointsForDimension1=[-5:5]  Table=tanh([-5:5])  InternalRulePriority=Speed  RndMeth=Simplest
  Rear tyre : MATLAB Function  TreatAsAtomicUnit=on
  camber vs wheel travel : Lookup_n-D  NumberOfTableDimensions=1  BreakpointsForDimension1=[-5:5]  Table=tanh([-5:5])  InternalRulePriority=Speed  RndMeth=Simplest
  Camber : Outport
  h_ground : Outport  Port=2
  wheel_travel_RL : Outport  Port=3
  wires:
  Delay One Step2/1 -> camber vs wheel travel/1
  Rear tyre/1(wheel_travel_RL) -> wheel_travel_RL/1, Delay One Step2/1, Delay One Step1/1, Delay One Step/1
  Delay One Step/1 -> IR vs wheel travel/1
  camber vs wheel travel/1 -> Camber/1
  Anti_squat vs wheel travel/1 -> Rear tyre/2(AS)
  IR vs wheel travel/1 -> Rear tyre/1(IR)
  Delay One Step1/1 -> Anti_squat vs wheel travel/1
  Rear tyre/2(h_ground) -> h_ground/1
  Fz/1 -> Rear tyre/4(Fz)
  delta_Fz/1 -> Rear tyre/5(delta_Fz)

== system Longitudinal_old/longitudinal dynamics/Kinematics/RR ==
  Fz : Inport
  delta_Fz : Inport  Port=2
  Anti_squat vs wheel travel : Lookup_n-D  NumberOfTableDimensions=1  BreakpointsForDimension1=[-5:5]  Table=tanh([-5:5])  InternalRulePriority=Speed  RndMeth=Simplest
  Delay One Step : Delay  DelayLength=1
  Delay One Step1 : Delay  DelayLength=1
  Delay One Step2 : Delay  DelayLength=1
  IR vs wheel travel : Lookup_n-D  NumberOfTableDimensions=1  BreakpointsForDimension1=[-5:5]  Table=tanh([-5:5])  InternalRulePriority=Speed  RndMeth=Simplest
  Rear tyre : MATLAB Function  TreatAsAtomicUnit=on
  camber vs wheel travel : Lookup_n-D  NumberOfTableDimensions=1  BreakpointsForDimension1=[-5:5]  Table=tanh([-5:5])  InternalRulePriority=Speed  RndMeth=Simplest
  Camber : Outport
  h_ground : Outport  Port=2
  delta_z_tyre_RR : Outport  Port=3
  wires:
  Delay One Step2/1 -> camber vs wheel travel/1
  Rear tyre/1(wheel_travel_RR) -> Delay One Step1/1, Delay One Step/1, Delay One Step2/1
  Delay One Step/1 -> IR vs wheel travel/1
  camber vs wheel travel/1 -> Camber/1
  Anti_squat vs wheel travel/1 -> Rear tyre/2(AS)
  IR vs wheel travel/1 -> Rear tyre/1(IR)
  Delay One Step1/1 -> Anti_squat vs wheel travel/1
  Rear tyre/2(h_ground) -> h_ground/1
  Fz/1 -> Rear tyre/4(Fz)
  delta_Fz/1 -> Rear tyre/5(delta_Fz)
  Rear tyre/4(delta_z_tyre_RR) -> delta_z_tyre_RR/1

== system Longitudinal_old/longitudinal dynamics original/Kinematics/Aeromaps ==
  h_front : Inport
  h_rear : Inport  Port=2
  Cx : Outport
  Cz : Outport  Port=2
  wires:
  h_front/1 -> Cx/1

== system Longitudinal_old/longitudinal dynamics original/Kinematics/Subsystem ==
  Fz : Inport
  Anti_squat vs wheel travel : Lookup_n-D  NumberOfTableDimensions=1  BreakpointsForDimension1=[-5:5]  Table=tanh([-5:5])  InternalRulePriority=Speed  RndMeth=Simplest
  Delay One Step : Delay  DelayLength=1
  Delay One Step1 : Delay  DelayLength=1
  Delay One Step2 : Delay  DelayLength=1
  IR vs wheel travel : Lookup_n-D  NumberOfTableDimensions=1  BreakpointsForDimension1=[-5:5]  Table=tanh([-5:5])  InternalRulePriority=Speed  RndMeth=Simplest
  MATLAB Function : MATLAB Function  TreatAsAtomicUnit=on
  XY Graph : Record  NumPorts=2.0  FileSettingsInternal="{\"entries\":[{\"content\":{\"excelSettings\":{\"content\":{},\"type\":\"Streamout.ExcelSettings\"},\"parquetSettings\":{\"content\":{},\"type\":\"Streamout.ParquetSettings\"}},\"type\":\"Streamout.FileSettingStorage\",\"uuid\":\"\"}],\"packageUris\":[\"http:\\/\\/schema.mathworks.com\\/mf0\\/streamout_blocks\\/R2020a\"],\"version\":\"1.0\"}"  FrameSettings=[0, 0]  Layout=[1 1]  SignalsInternal="{\"entries\":[{\"content\":{\"signals\":[{\"content\":{\"blockPath\":[],\"dimensions\":[1],\"domain\":\"\",\"lineColor\":\"#a2142f\",\"plots\":[ 1 ],\"port\":1,\"signalID\":1,\"signalName\":\"XY Graph:1\"},\"type\":\"RecordBlkView.Signal\",\"uuid\":\"\"},{\"content\":{\"blockPath\":[],\"dimensions\":[1],\"domain\":\"\",\"lineColor\":\"#139fff\",\"plots\":[ 1 ],\"port\":2,\"signalID\":2,\"signalName\":\"XY Graph:2\"},\"type\":\"RecordBlkView.Signal\",\"uuid\":\"\"}]},\"type\":\"RecordBlkView.InputSignals\",\"uuid\":\"\"}],\"packageUris\":[\"http:\\/\\/schema.mathworks.com\\/mf0\\/streamout_blocks\\/R2020a\"],\"version\":\"1.0\"}"  VisualizationBindings="{\"xyplotplugin\":{\"info\":[{\"series\":[{\"bindingParametersList\":[{\"parameter\":\"X-Axis\",\"signalID\":1,\"signalName\":\"XY Graph:1\"},{\"parameter\":\"Y-Axis\",\"signalID\":2,\"signalName\":\"XY Graph:2\"}],\"seriesID\":0}],\"subplotID\":1}]}}"  CompatibilityTag=XY
  camber vs wheel travel : Lookup_n-D  NumberOfTableDimensions=1  BreakpointsForDimension1=[-5:5]  Table=tanh([-5:5])  InternalRulePriority=Speed  RndMeth=Simplest
  Camber : Outport
  h_ground : Outport  Port=2
  wires:
  Delay One Step2/1 -> camber vs wheel travel/1
  MATLAB Function/1(wheel_travel) -> Delay One Step2/1, Delay One Step1/1, Delay One Step/1
  Delay One Step/1 -> IR vs wheel travel/1
  camber vs wheel travel/1 -> Camber/1
  Anti_squat vs wheel travel/1 -> MATLAB Function/2(AS)
  IR vs wheel travel/1 -> MATLAB Function/1(IR)
  Delay One Step1/1 -> Anti_squat vs wheel travel/1
  MATLAB Function/2(h_ground) -> h_ground/1
  Fz/1 -> MATLAB Function/4(Fz)

== system Longitudinal_old/longitudinal dynamics original/Kinematics/Subsystem1 ==
  Fz : Inport
  Anti_squat vs wheel travel : Lookup_n-D  NumberOfTableDimensions=1  BreakpointsForDimension1=[-5:5]  Table=tanh([-5:5])  InternalRulePriority=Speed  RndMeth=Simplest
  Delay One Step : Delay  DelayLength=1
  Delay One Step1 : Delay  DelayLength=1
  Delay One Step2 : Delay  DelayLength=1
  IR vs wheel travel : Lookup_n-D  NumberOfTableDimensions=1  BreakpointsForDimension1=[-5:5]  Table=tanh([-5:5])  InternalRulePriority=Speed  RndMeth=Simplest
  MATLAB Function : MATLAB Function  TreatAsAtomicUnit=on
  camber vs wheel travel : Lookup_n-D  NumberOfTableDimensions=1  BreakpointsForDimension1=[-5:5]  Table=tanh([-5:5])  InternalRulePriority=Speed  RndMeth=Simplest
  Camber : Outport
  h_ground : Outport  Port=2
  wires:
  Delay One Step2/1 -> camber vs wheel travel/1
  MATLAB Function/1(wheel_travel) -> Delay One Step2/1, Delay One Step1/1, Delay One Step/1
  Delay One Step/1 -> IR vs wheel travel/1
  camber vs wheel travel/1 -> Camber/1
  Anti_squat vs wheel travel/1 -> MATLAB Function/2(AS)
  IR vs wheel travel/1 -> MATLAB Function/1(IR)
  Delay One Step1/1 -> Anti_squat vs wheel travel/1
  MATLAB Function/2(h_ground) -> h_ground/1
  Fz/1 -> MATLAB Function/3(Fz)

== system Longitudinal_old/longitudinal dynamics original/Kinematics/Subsystem2 ==
  Fz : Inport
  Anti_squat vs wheel travel : Lookup_n-D  NumberOfTableDimensions=1  BreakpointsForDimension1=[-5:5]  Table=tanh([-5:5])  InternalRulePriority=Speed  RndMeth=Simplest
  Delay One Step : Delay  DelayLength=1
  Delay One Step1 : Delay  DelayLength=1
  Delay One Step2 : Delay  DelayLength=1
  IR vs wheel travel : Lookup_n-D  NumberOfTableDimensions=1  BreakpointsForDimension1=[-5:5]  Table=tanh([-5:5])  InternalRulePriority=Speed  RndMeth=Simplest
  MATLAB Function : MATLAB Function  TreatAsAtomicUnit=on
  camber vs wheel travel : Lookup_n-D  NumberOfTableDimensions=1  BreakpointsForDimension1=[-5:5]  Table=tanh([-5:5])  InternalRulePriority=Speed  RndMeth=Simplest
  Camber : Outport
  h_ground : Outport  Port=2
  wires:
  Delay One Step2/1 -> camber vs wheel travel/1
  MATLAB Function/1(wheel_travel) -> Delay One Step2/1, Delay One Step1/1, Delay One Step/1
  Delay One Step/1 -> IR vs wheel travel/1
  camber vs wheel travel/1 -> Camber/1
  Anti_squat vs wheel travel/1 -> MATLAB Function/2(AS)
  IR vs wheel travel/1 -> MATLAB Function/1(IR)
  Delay One Step1/1 -> Anti_squat vs wheel travel/1
  MATLAB Function/2(h_ground) -> h_ground/1
  Fz/1 -> MATLAB Function/3(Fz)

== system Longitudinal_old/longitudinal dynamics original/Kinematics/Subsystem3 ==
  Fz : Inport
  Anti_squat vs wheel travel : Lookup_n-D  NumberOfTableDimensions=1  BreakpointsForDimension1=[-5:5]  Table=tanh([-5:5])  InternalRulePriority=Speed  RndMeth=Simplest
  Delay One Step : Delay  DelayLength=1
  Delay One Step1 : Delay  DelayLength=1
  Delay One Step2 : Delay  DelayLength=1
  IR vs wheel travel : Lookup_n-D  NumberOfTableDimensions=1  BreakpointsForDimension1=[-5:5]  Table=tanh([-5:5])  InternalRulePriority=Speed  RndMeth=Simplest
  MATLAB Function : MATLAB Function  TreatAsAtomicUnit=on
  camber vs wheel travel : Lookup_n-D  NumberOfTableDimensions=1  BreakpointsForDimension1=[-5:5]  Table=tanh([-5:5])  InternalRulePriority=Speed  RndMeth=Simplest
  Camber : Outport
  h_ground : Outport  Port=2
  wires:
  Delay One Step2/1 -> camber vs wheel travel/1
  MATLAB Function/1(wheel_travel) -> Delay One Step2/1, Delay One Step1/1, Delay One Step/1
  Delay One Step/1 -> IR vs wheel travel/1
  camber vs wheel travel/1 -> Camber/1
  Anti_squat vs wheel travel/1 -> MATLAB Function/2(AS)
  IR vs wheel travel/1 -> MATLAB Function/1(IR)
  Delay One Step1/1 -> Anti_squat vs wheel travel/1
  MATLAB Function/2(h_ground) -> h_ground/1
  Fz/1 -> MATLAB Function/3(Fz)

== matlab function Longitudinal_old/longitudinal dynamics/Min Fx solver/RR ==
  data: Fx_ICE input; Fx_RR output; Fx_tyre input; delta_Fx_RR output
function [Fx_RR, delta_Fx_RR] = fcn(Fx_ICE, Fx_tyre)

% add delta Fx for each tyre

if Fx_ICE<Fx_tire
    Fx_RR = Fx_ICE;
else 
    Fx_RR = Fx_tire;
    delta_Fx_RR = Fx_ICE - Fx_tire;
end

== matlab function Longitudinal_old/longitudinal dynamics/Kinematics/FR/Front tyre ==
  data: wheel_travel_FR output; IR input; AS input; AD input; h_ground output; Fz input; delta_Fz input; jounce_front output
function [wheel_travel_FR, h_ground, jounce_front]    = kinematics(IR, AS, AD, Fz, delta_Fz)

delta_z_tyre = Fz / kz_tyre; % tyre vertical stiffness - kz_tyre - for front and rear tyres, look at buses
k_spring_ground = (k_spring * IR^2);

if a > 0 % under acceleration
    delta_z_spring_front = Fz / k_spring_ground; % front axle
else % under braking
    delta_z_spring_front = (Fz - delta_Fz) / k_spring_ground + delta_Fz * ((1-AD)/k_spring_ground) ; % front axle
end

%wheel center movement only due to spring deflection at ground. 
%to be used in the kineamtics block (camber, antidive, ir,...)
wheel_travel_front = delta_z_spring_front - z0_spring_front; % if negative it is bounce

%to be used to find the new height of the car from the ground
jounce_front = delta_z_tyre + delta_z_spring_front - z0_front;
h_ground_front = h0_ground_front - jounce_front;

== matlab function Longitudinal_old/Tyres/Front Left ==
  data: tyre input; SR input; Fx_FL output; Fz input; camber input
function Fx_FL = fcn(tyre,SR,Fz,camber)

% PAC2002 puro longitudinale (Fx vs k)

     Fz0 = tyre.Fz0;
     if Fz0 == 0, Fz0 = max(1, Fz); end
    dfz = (Fz - Fz0)/Fz0;

    pi0 = tyre.pi0;  % Pa nominale
    dpi = (tyre.pressure.front - pi0)/pi0;
    
    Cx1 = tyre.Cx1;
    Dx1 = tyre.Dx1;
    Dx2 = tyre.Dx2;
    Dx3 = tyre.Dx3;
    Ex1 = tyre.Ex1;
    Ex2 = tyre.Ex2;
    Ex3 = tyre.Ex3;
    Ex4 = tyre.Ex4;
    Kx1 = tyre.Kx1;
    Kx2 = tyre.Kx2;
    Kx3 = tyre.Kx3;
    Hx1 = tyre.Hx1;
    Hx2 = tyre.Hx2;
    Vx1 = tyre.Vx1;
    Vx2 = tyre.Vx2;
    px1 = tyre.px1;
    px2 = tyre.px2;
    px3 = tyre.px3;
    px4 = tyre.px4;
    lmux = tyre.lmux;

    gamma = camber*pi/180;
    mu = (Dx1 + Dx2*dfz) * (1 - Dx3*(gamma^2)) * (1 + px3*dpi + px4*dpi^2)*lmux;
    % mu = 1.4;

    D = mu * Fz;
    C = Cx1;
    K = Fz * (Kx1 + Kx2*dfz) * exp(Kx3*dfz) * (1 + px1*dpi + px2*dpi^2);
    B = K / (C*D + eps);

    SH = Hx1 + Hx2*dfz;
    SR  = SR + SH;

    E  = (Ex1 + Ex2*dfz + Ex3*dfz^2) * (1 - Ex4*sign(SR));
    SV = Fz * (Vx1 + Vx2*dfz);

    Fx0 = D * sin( C * atan( B*SR - E*(B*SR - atan(B*SR)) ) );
    Fx_FL = Fx0 + SV;

== matlab function Longitudinal_old/longitudinal dynamics/Kinematics/RR/Rear tyre ==
  data: wheel_travel_RR output; IR input; AS input; AD input; h_ground output; Fz input; delta_Fz input; jounce_rear output; delta_z_tyre_RR output
function [wheel_travel_RR, h_ground, jounce_rear, delta_z_tyre_RR]      = kinematics(IR, AS, AD, Fz, delta_Fz)

delta_z_tyre_RR = Fz / kz_tyre; % tyre vertical stiffness - kz_tyre - for front and rear tyres, look at buses
k_spring_ground = (k_spring * IR^2);

if a > 0 % under acceleration
    delta_z_spring_rear = (Fz - delta_Fz) / k_spring_ground + delta_Fz * ((1-AS)/k_spring_ground) ; % rear axle
else % under braking
    delta_z_spring_rear = Fz / k_spring_ground; % rear axle
end

wheel_travel_rear = delta_z_spring_rear - z0_spring_rear; % if negative it is bounce

jounce_rear = delta_z_tyre_RR + delta_z_spring_rear - z0_rear;

% h_ground_front = ;
% h_ground_rear = ;

% h_ground = delta_z - z_0;
% wheel_travel =  h_ground - delta_z_tyre;

% does the AS contribute to less tyre deflection or just smaller spring
% deflection?
% static height - how do we take it - when wheels are on the ground

== matlab function Longitudinal_old/longitudinal dynamics/Subsystem/RR ==
  data: delta_Fx_rear input; w_dot_tyre_RR output; delta_z_tyre input
function w_dot_tyre_RR  = fcn(delta_Fx_rear, delta_z_tyre)

% use bus for all tyres

w_dot_tyre_rear = delta_Fx_rear * (R - delta_z_tyre_rear) * eta_pwt / J_r;

== matlab function Longitudinal_old/longitudinal dynamics/Kinematics/FL/Front tyre ==
  data: wheel_travel_FL output; IR input; AS input; AD input; h_ground output; Fz input; delta_Fz input; jounce_front output
function [wheel_travel_FL, h_ground, jounce_front]    = kinematics(IR, AS, AD, Fz, delta_Fz)

delta_z_tyre = Fz / kz_tyre; % tyre vertical stiffness - kz_tyre - for front and rear tyres, look at buses
k_spring_ground = (k_spring * IR^2);

if a > 0 % under acceleration
    delta_z_spring_front = Fz / k_spring_ground; % front axle
else % under braking
    delta_z_spring_front = (Fz - delta_Fz) / k_spring_ground + delta_Fz * ((1-AD)/k_spring_ground) ; % front axle
end

%wheel center movement only due to spring deflection at ground. 
%to be used in the kineamtics block (camber, antidive, ir,...)
wheel_travel_front = delta_z_spring_front - z0_spring_front; % if negative it is bounce

%to be used to find the new height of the car from the ground
jounce_front = delta_z_tyre + delta_z_spring_front - z0_front;
h_ground_front = h0_ground_front - jounce_front;

== matlab function Longitudinal_old/longitudinal dynamics/Subsystem/FR ==
  data: delta_Fx_front input; delta_z_tyre input; w_dot_tyre_FR output
function w_dot_tyre_FR  = fcn(delta_Fx_front, delta_z_tyre)

w_dot_tyre_front = delta_Fx_front * (R - delta_z_tyre_front) * eta_pwt / J_f;

== matlab function Longitudinal_old/longitudinal dynamics original/Kinematics/Subsystem1/MATLAB Function ==
  data: wheel_travel output; IR input; AS input; h_ground output; Fz input
function [wheel_travel, h_ground]    = kinematics(IR, AS, Fz)

delta_z_tyre = Fz / kz_tyre; % tyre vertical  stiffness - kz_tyre
1 / k_eq = 1 /(k_spring * IR) + 1/ kz_tyre;
delta_z = Fz * ((1-AS)/k_eq); % AS - anti-squat spring - ground travel vs chassis
h_ground = delta_z - z_0;
wheel_travel =  h_ground - delta_z_tyre;

== matlab function Longitudinal_old/longitudinal dynamics original/Kinematics/Subsystem2/MATLAB Function ==
  data: wheel_travel output; IR input; AS input; h_ground output; Fz input
function [wheel_travel, h_ground]    = kinematics(IR, AS, Fz)

delta_z_tyre = Fz / kz_tyre; % tyre vertical stiffness- kz_tyre
1 / k_eq = 1 /(k_spring * IR) + 1/ kz_tyre;
delta_z = Fz * ((1-AS)/k_eq); % AS - anti-squat spring - ground travel vs chassis
h_ground = delta_z - z_0;
wheel_travel =  h_ground - delta_z_tyre;

== matlab function Longitudinal_old/longitudinal dynamics original/Kinematics/Subsystem3/MATLAB Function ==
  data: wheel_travel output; IR input; AS input; h_ground output; Fz input
function [wheel_travel, h_ground]    = kinematics(IR, AS, Fz)

delta_z_tyre = Fz / kz_tyre; % tyre vertical stiffness - kz_tyre
1 / k_eq = 1 /(k_spring * IR) + 1/ kz_tyre;
delta_z = Fz * ((1-AS)/k_eq); % AS - anti-squat spring - ground travel vs chassis
h_ground = delta_z - z_0;
wheel_travel =  h_ground - delta_z_tyre;

== matlab function Longitudinal_old/longitudinal dynamics original/MATLAB Function ==
  data: delta_Fx_rear input; w_dot_tyre_rear output; delta_z_tyre input; w_dot_tyre_front output
function [w_dot_tyre_rear, w_dot_tyre_front] = fcn(delta_Fx_rear, delta_z_tyre)

% use bus for all tyres

w_dot_tyre_rear = delta_Fx_rear * (R - delta_z_tyre_rear) * eta_pwt / J_r;
w_dot_tyre_front = delta_Fx_front * (R - delta_z_tyre_front) * eta_pwt / J_f;

== matlab function Longitudinal_old/longitudinal dynamics original/Kinematics/Subsystem/MATLAB Function ==
  data: wheel_travel output; IR input; AS input; AD input; h_ground output; Fz input; delta_Fz input; jounce_rear output; jounce_front output
function [wheel_travel, h_ground, jounce_rear, jounce_front]    = kinematics(IR, AS, AD, Fz, delta_Fz)

delta_z_tyre = Fz / kz_tyre; % tyre vertical stiffness - kz_tyre - for front and rear tyres, look at buses
k_spring_ground = (k_spring * IR^2);

if a > 0 % under acceleration
    delta_z_spring_rear = (Fz - delta_Fz) / k_spring_ground + delta_Fz * ((1-AS)/k_spring_ground) ; % rear axle
    delta_z_spring_front = Fz / k_spring_ground; % front axle
else % under braking
    delta_z_spring_rear = Fz / k_spring_ground; % rear axle
    delta_z_spring_front = (Fz - delta_Fz) / k_spring_ground + delta_Fz * ((1-AD)/k_spring_ground) ; % front axle
end

wheel_travel_rear = delta_z_spring_rear - z0_spring_rear; % if negative it is bounce
wheel_travel_front = delta_z_spring_front - z0_spring_front; % if negative it is bounce

jounce_rear = delta_z_tyre + delta_z_spring_rear - z0_rear;
jounce_front = delta_z_tyre + delta_z_spring_front - z0_front;

h_ground_front = ;
h_ground_rear = ;

% h_ground = delta_z - z_0;
% wheel_travel =  h_ground - delta_z_tyre;

% does the AS contribute to less tyre deflection or just smaller spring
% deflection?
% static height - how do we take it - when wheels are on the ground

== matlab function Longitudinal_old/longitudinal dynamics original/MATLAB Function2 ==
  data: Fz_FL output; a input; Fz_RR output; Fz_RL output; Fz_FR output; delta_Fz output; v input
function [Fz_FL, Fz_RR, Fz_RL, Fz_FR, delta_Fz] = fx_equilibrium(a, v)

Downforce = 0.5 * rho * Cz * A * v ^ 2; % downforce
Drag = 0.5 * rho * Cx * A * v ^2; % drag
M_aero = Drag * (h_cp - h_cog) - Downforce * (lf-x_cp);

delta_Fz = m * a * h_cog / wb + Drag * h_cog / wb + M_aero / wb;

Fz_front = -(m * a + Drag) * h_cog / wb + ( m * g - Downforce ) * (lr -delta) / wb - M_aero / wb - J_f * a / (R * wb);

Fz_FR = Fz_front / 2;
Fz_FL = Fz_FR;

Fz_front = (m * a + Drag) * h_cog / wb + ( m * g - Downforce ) * (lf + delta) / wb + M_aero / wb + J_r * a / (R * wb);

Fz_RR = Fz_rear / 2;
Fz_RL = Fz_RR;

== matlab function Longitudinal_old/longitudinal dynamics original/Min Fx calculator ==
  data: Fx_ICE_RR input; Fx_FR output; Fx_ICE_RL input; Fx_EM_FR input; Fx_EM_FL input; Fx_tyre_FR input; Fx_tyre_FL input; Fx_tyre_RR input; Fx_tyre_RL input; Fx_RR output; Fx_RL output; Fx_FL output; delta_Fx output
function [Fx_FR, Fx_RR, Fx_RL, Fx_FL, delta_Fx] = fcn(Fx_ICE_RR, Fx_ICE_RL, Fx_EM_FR, Fx_EM_FL, Fx_tyre_FR, Fx_tyre_FL, Fx_tyre_RR, Fx_tyre_RL)

% add delta Fx for each tyre

if Fx_ICE<Fx_tire
    Fx = Fx_ICE;
else 
    Fx = Fx_tire;
    delta_Fx = Fx_ICE - Fx_tire;
end

Fx_total = % Fill this

== matlab function Longitudinal_old/longitudinal dynamics original/Subsystem/MATLAB Function ==
  data: Fz input; Fx output; T input; J input
function Fx = fcn(Fz, T, J)

Fx = (T - Fz * delta - J * a / R) / R ; % J - parameter for each tyre - J_f & J_r

== matlab function Longitudinal_old/longitudinal dynamics/Fx powertrain calculation/RR ==
  data: Fz input; Fx_ICE_RR output; T input
function Fx_ICE_RR = fcn(Fz, T)

Fx_ICE_RR = (T - Fz * delta - J_r * a / R) / R ; % J - parameter for each tyre - J_f & J_r

== matlab function Longitudinal_old/longitudinal dynamics/Fx powertrain calculation/FR ==
  data: Fz input; Fx_EM_FR output; T input
function Fx_EM_FR = fcn(Fz, T)

Fx_EM_FR = (T - Fz * delta - J_f * a / R) / R ; % J - parameter for each tyre - J_f & J_r

== matlab function Longitudinal_old/longitudinal dynamics/Fx powertrain calculation/RL ==
  data: Fz input; Fx_ICE_RL output; T input
function Fx_ICE_RL = fcn(Fz, T)

Fx_ICE_RL = (T - Fz * delta - J_r * a / R) / R ; % J - parameter for each tyre - J_f & J_r

== matlab function Longitudinal_old/longitudinal dynamics/Min Fx solver/RL ==
  data: Fx_ICE input; Fx_RL output; Fx_tyre input; delta_Fx_RL output
function [Fx_RL, delta_Fx_RL] = fcn(Fx_ICE, Fx_tyre)

% add delta Fx for each tyre

if Fx_ICE<Fx_tire
    Fx_RL = Fx_ICE;
else 
    Fx_RL = Fx_tire;
    delta_Fx_RL = Fx_ICE - Fx_tire;
end
